simulink model "six_dof_2018a"  (R2018a)
settings: Solver=VariableStepAuto  StartTime=0.0  StopTime=TF  RelTol=1e-3
values from neighbouring files (symbols this model uses):
  x_init = [ ... (first row only)    [F16_model_test.m]
undefined symbols (not defined in the file or in its folder): F16_aerodynamics, F16_propulsion, gravity_model, intermediate_func, nonlinear_6DOF
settings Model: Creator=parth  LastModifiedBy=parth
settings DataIOCC: ReturnWorkspaceOutputs=on
settings SFSimCC: SimUseLocalCustomCode=on
settings RTWCC: RTWUseLocalCustomCode=on

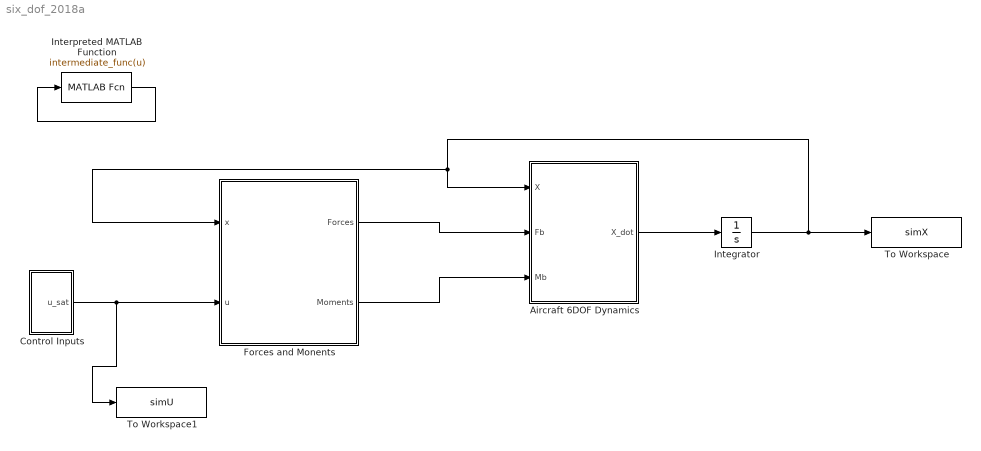
== system six_dof_2018a ==
  Aircraft 6DOF Dynamics : Subsystem
  Control Inputs : Subsystem
  Forces and Monents : Subsystem
  Integrator : Integrator  InitialCondition=x_init
  Interpreted MATLAB Function : MATLABFcn  MATLABFcn=intermediate_func(u)
  To Workspace : ToWorkspace  VariableName=simX  SaveFormat=Timeseries  SampleTime=-1
  To Workspace1 : ToWorkspace  VariableName=simU  SaveFormat=Timeseries  SampleTime=-1
  wires:
  Aircraft 6DOF Dynamics/1(X_dot) -> Integrator/1
  Forces and Monents/1(Forces) -> Aircraft 6DOF Dynamics/2(Fb)
  Forces and Monents/2(Moments) -> Aircraft 6DOF Dynamics/3(Mb)
  Control Inputs/1(u_sat) -> Forces and Monents/2(u), To Workspace1/1
  Integrator/1 -> Forces and Monents/1(x), Aircraft 6DOF Dynamics/1(X), To Workspace/1
  Interpreted MATLAB Function/1 -> Interpreted MATLAB Function/1

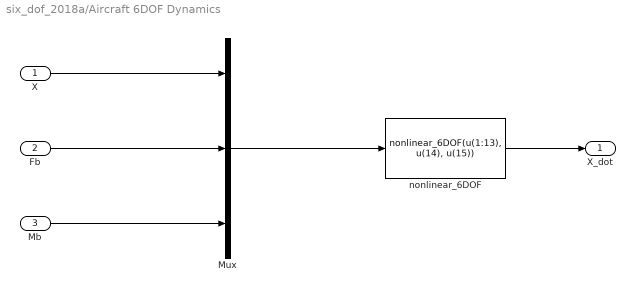
== system six_dof_2018a/Aircraft 6DOF Dynamics ==
  X : Inport
  Fb : Inport  Port=2
  Mb : Inport  Port=3
  Mux : Mux  Inputs=3
  nonlinear_6DOF : MATLABFcn  MATLABFcn=nonlinear_6DOF(u(1:13), u(14), u(15))  OutputDimensions=13
  X_dot : Outport
  wires:
  Mb/1 -> Mux/3
  Fb/1 -> Mux/2
  nonlinear_6DOF/1 -> X_dot/1
  Mux/1 -> nonlinear_6DOF/1
  X/1 -> Mux/1

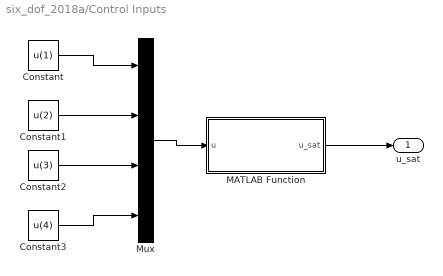
== system six_dof_2018a/Control Inputs ==
  Constant : Constant  Value=u(1)
  Constant1 : Constant  Value=u(2)
  Constant2 : Constant  Value=u(3)
  Constant3 : Constant  Value=u(4)
  MATLAB Function : MATLAB Function  TreatAsAtomicUnit=on
  Mux : Mux
  u_sat : Outport
  wires:
  Constant/1 -> Mux/1
  Constant3/1 -> Mux/4
  MATLAB Function/1(u_sat) -> u_sat/1
  Constant2/1 -> Mux/3
  Constant1/1 -> Mux/2
  Mux/1 -> MATLAB Function/1(u)

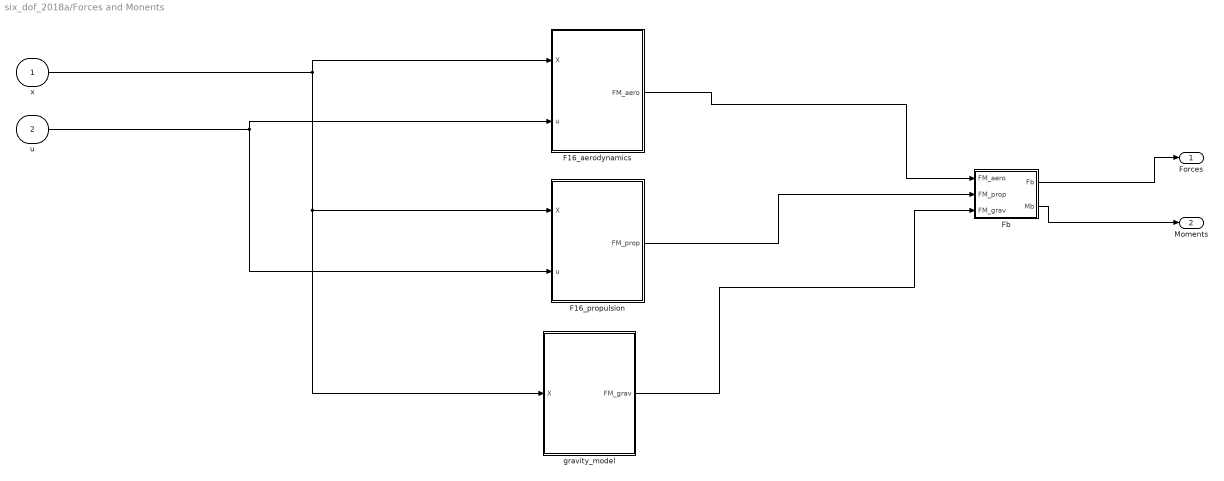
== system six_dof_2018a/Forces and Monents ==
  x : Inport
  u : Inport  Port=2
  F16_aerodynamics : Subsystem
  F16_propulsion : Subsystem
  Fb : Subsystem
  gravity_model : Subsystem
  Forces : Outport
  Moments : Outport  Port=2
  wires:
  Fb/2(Mb) -> Moments/1
  Fb/1(Fb) -> Forces/1
  F16_aerodynamics/1(FM_aero) -> Fb/1(FM_aero)
  gravity_model/1(FM_grav) -> Fb/3(FM_grav)
  F16_propulsion/1(FM_prop) -> Fb/2(FM_prop)
  x/1 -> F16_aerodynamics/1(X), gravity_model/1(X), F16_propulsion/1(X)
  u/1 -> F16_aerodynamics/2(u), F16_propulsion/2(u)

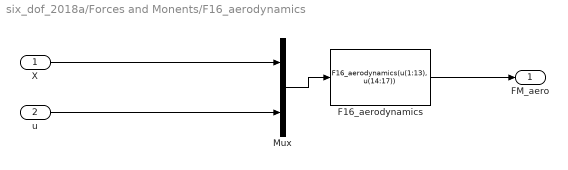
== system six_dof_2018a/Forces and Monents/F16_aerodynamics ==
  X : Inport
  u : Inport  Port=2
  F16_aerodynamics : MATLABFcn  MATLABFcn=F16_aerodynamics(u(1:13), u(14:17))  OutputDimensions=6
  Mux : Mux  Inputs=2
  FM_aero : Outport
  wires:
  Mux/1 -> F16_aerodynamics/1
  u/1 -> Mux/2
  X/1 -> Mux/1
  F16_aerodynamics/1 -> FM_aero/1

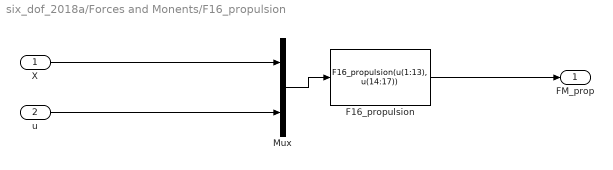
== system six_dof_2018a/Forces and Monents/F16_propulsion ==
  X : Inport
  u : Inport  Port=2
  F16_propulsion : MATLABFcn  MATLABFcn=F16_propulsion(u(1:13), u(14:17))  OutputDimensions=6
  Mux : Mux  Inputs=2
  FM_prop : Outport
  wires:
  Mux/1 -> F16_propulsion/1
  u/1 -> Mux/2
  X/1 -> Mux/1
  F16_propulsion/1 -> FM_prop/1

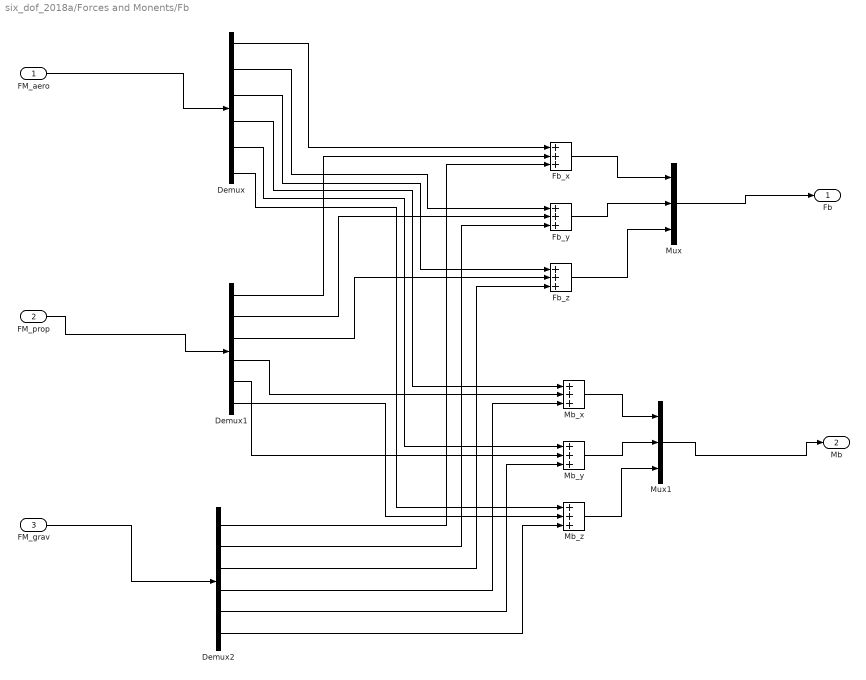
== system six_dof_2018a/Forces and Monents/Fb ==
  FM_aero : Inport
  FM_prop : Inport  Port=2
  FM_grav : Inport  Port=3
  Demux : Demux  Outputs=6
  Demux1 : Demux  Outputs=6
  Demux2 : Demux  Outputs=6
  Fb_x : Sum  Inputs=+++
  Fb_y : Sum  Inputs=+++
  Fb_z : Sum  Inputs=+++
  Mb_x : Sum  Inputs=+++
  Mb_y : Sum  Inputs=+++
  Mb_z : Sum  Inputs=+++
  Mux : Mux  Inputs=3
  Mux1 : Mux  Inputs=3
  Fb : Outport
  Mb : Outport  Port=2
  wires:
  Demux1/2 -> Fb_y/2
  Demux/2 -> Fb_y/1
  Fb_x/1 -> Mux/1
  Demux/3 -> Fb_z/1
  Demux1/3 -> Fb_z/2
  Demux2/3 -> Fb_z/3
  Fb_z/1 -> Mux/3
  Demux1/1 -> Fb_x/2
  Demux2/1 -> Fb_x/3
  Fb_y/1 -> Mux/2
  Demux2/2 -> Fb_y/3
  Demux/1 -> Fb_x/1
  Mb_y/1 -> Mux1/2
  Mb_x/1 -> Mux1/1
  Mb_z/1 -> Mux1/3
  Demux/4 -> Mb_x/1
  Demux1/4 -> Mb_x/2
  Demux2/4 -> Mb_x/3
  Demux/5 -> Mb_y/1
  Demux1/5 -> Mb_y/2
  Demux2/5 -> Mb_y/3
  Demux/6 -> Mb_z/1
  Demux1/6 -> Mb_z/2
  Demux2/6 -> Mb_z/3
  FM_aero/1 -> Demux/1
  FM_prop/1 -> Demux1/1
  FM_grav/1 -> Demux2/1
  Mux/1 -> Fb/1
  Mux1/1 -> Mb/1

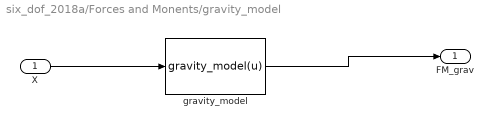
== system six_dof_2018a/Forces and Monents/gravity_model ==
  X : Inport
  gravity_model : MATLABFcn  MATLABFcn=gravity_model(u)  OutputDimensions=6
  FM_grav : Outport
  wires:
  X/1 -> gravity_model/1
  gravity_model/1 -> FM_grav/1

== matlab function six_dof_2018a/Control Inputs/MATLAB Function ==
  data: u input; u_sat output
function u_sat = control_saturation(u)
% saturate controls
% u = [delta_T, delta_e, delta_a, delta_r]

u_sat = zeros(4,1);

u_sat(1) = bound_function(u(1), 0, 1);
u_sat(2) = bound_function(u(2), -0.4363, 0.4363); % -25 to 25 deg
u_sat(3) = bound_function(u(3), -0.3752, 0.3752); % -21.5 to 21.5 deg
u_sat(4) = bound_function(u(4), -0.5236, 0.5236); % -30 to 30 deg

end
